simulink model "Project2024_Group3"  (R2023b)
settings: Solver=VariableStepAuto  StartTime=0.0  StopTime=25  RelTol=1e-3
InitFcn:
  | clear;
StopFcn:
  | plot_results(out);
  | compute_indices(out);
values from neighbouring files (symbols this model uses):
  D = 3500    [Project2024_params_Group3.m]
  m = -0.09    [Project2024_params_Group3.m]
  MAP_eq = 90    [Project2024_params_Group3.m]    (also in compute_indices.m = mean(MAP_data(pre_infusion_indices)))
  RAP = 5    [Project2024_params_Group3.m]
  SV = 0.097    [Project2024_params_Group3.m]
  T = 10    [Project2024_params_Group3.m]
settings Model: Creator=jamesyeh  LastModifiedBy=jamesyeh
settings ModelReferenceCC: ModelDependencies=Project2024_params_Group3.m

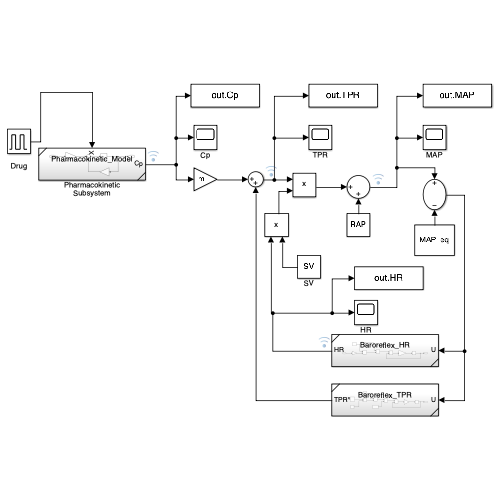
[thumbnail: Simulink's stored preview of the top-level diagram]
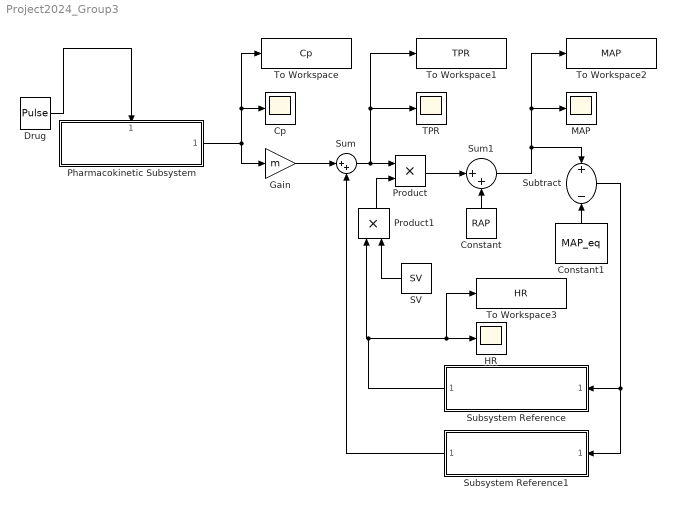
== system Project2024_Group3 ==
  " Drug" : DiscretePulseGenerator  PulseType=Time based  Amplitude=D/T  Period=1e6  PulseWidth=10/1e6*100  PhaseDelay=1
  Constant : Constant  Value=RAP
  Constant1 : Constant  Value=MAP_eq
  Cp : Scope
  Gain : Gain  Gain=m
  HR : Scope
  MAP : Scope
  Pharmacokinetic Subsystem : Subsystem  ReferencedSubsystem=Pharmacokinetic_Model
      settings: PortSchema="{\"entries\":[{\"content\":{\"sides\":[{\"content\":{},\"type\":\"ConnectorPlacement.EquallySpacedRectSide\",\"uuid\":\"724ed912-986b-4240-841d-995132398956\"},{\"content\":{\"connectorIds\":[\"Out1\"],\"side\":\"RIGHT\"},\"type\":\"ConnectorPlacement.EquallySpacedRectSide\",\"uuid\":\"17b6dfd6-0df0-409a-9a6c-db7d93797c4e\"},{\"content\":{\"connectorIds\":[\"In1\"],\"side\":\"TOP\"},\"type\":\"ConnectorPlacement.EquallySpacedRectSide\",\"uuid\":\"f9d6e6fd-7e2f-4a54-85f1-4c033b63db6c\"}]},\"type\":\"ConnectorPlacement.EquallySpacedConnector\",\"uuid\":\"04ba1d6e-1f4b-4b43-a90a-d746b1ef254c\"}],\"packageUris\":[\"http://schema.mathworks.com/mf0/Connector/R2020b\"],\"version\":\"1.0\"}"
  Product : Product
  Product1 : Product
  SV : Constant  Value=SV
  Subsystem Reference : Subsystem  ReferencedSubsystem=Baroreflex_HR
  Subsystem Reference1 : Subsystem  ReferencedSubsystem=Baroreflex_TPR
  Subtract : Sum  Inputs=+-
  Sum : Sum  Inputs=|++
  Sum1 : Sum  Inputs=|++
  TPR : Scope
  To Workspace : ToWorkspace  VariableName=Cp  SaveFormat=Structure With Time  SampleTime=-1
  To Workspace1 : ToWorkspace  VariableName=TPR  SaveFormat=Structure With Time  SampleTime=-1
  To Workspace2 : ToWorkspace  VariableName=MAP  SaveFormat=Structure With Time  SampleTime=-1
  To Workspace3 : ToWorkspace  VariableName=HR  SaveFormat=Structure With Time  SampleTime=-1
  wires:
  Constant/1 -> Sum1/2
  Product/1 -> Sum1/1
  Gain/1 -> Sum/1
  Sum/1 -> To Workspace1/1, TPR/1, Product/1
  Pharmacokinetic Subsystem/1 -> To Workspace/1, Cp/1, Gain/1
  " Drug"/1 -> Pharmacokinetic Subsystem/1
  Sum1/1 -> To Workspace2/1, MAP/1, Subtract/1
  Constant1/1 -> Subtract/2
  Subtract/1 -> Subsystem Reference1/1, Subsystem Reference/1
  Subsystem Reference/1 -> Product1/1, To Workspace3/1, HR/1
  SV/1 -> Product1/2
  Product1/1 -> Product/2
  Subsystem Reference1/1 -> Sum/2
